simulink model "Vehicle_Dynamic_sim_V0605"  (R2017a)
settings: Solver=FixedStepAuto  StartTime=0.0  StopTime=50  FixedStep=0.001  RelTol=1e-3  EnableMultiTasking=on
PreLoadFcn:
  | load CarSim_FE4_2.mat
  | load Vehicle_information_test_0525_2017.mat
  | load CarSim0524.mat
values from neighbouring files (symbols this model uses):
  a = [(-2/tau - 1/tau_0) 1/tau 1/tau; 1/tau -2/tau 1/tau; 1/tau 1/tau -2/tau]    [MAE_272A_HW2_Q1a.m]    (also in Vehicle_Dynamic_main.m = 0.624; Vehicle_Dynamic_main_V0.m = 0.624; Vehicle_Dynamic_main_V01.m = 0.624; Vehicle_Dynamic_main_V0605.m = 0.624)
  aa = weight_front*wheelbase    (= 0.7875)    [Vehicle_Dynamic_main.m]    (also in Vehicle_Dynamic_main_V0.m; Vehicle_Dynamic_main_V01.m; Vehicle_Dynamic_main_V0605.m; Vehicle_Dynamic_main_V0629.m)
  b = [1/A 0; 0 1/A; 0 0]    [MAE_272A_HW2_Q1a.m]    (also in Vehicle_Dynamic_main.m = 0.624; Vehicle_Dynamic_main_V0.m = 0.624; Vehicle_Dynamic_main_V01.m = 0.624; Vehicle_Dynamic_main_V0605.m = 0.624)
  bb = weight_rear*wheelbase    (= 0.7875)    [Vehicle_Dynamic_main.m]    (also in Vehicle_Dynamic_main_V0.m; Vehicle_Dynamic_main_V01.m; Vehicle_Dynamic_main_V0605.m; Vehicle_Dynamic_main_V0629.m)
  g = 9.81    [Vehicle_Dynamic_main.m]    (also in Vehicle_Dynamic_main_V0.m; Vehicle_Dynamic_main_V01.m; Vehicle_Dynamic_main_V0605.m; Vehicle_Dynamic_main_V0629.m)
  hf = 0.20729    [Vehicle_Dynamic_main.m]    (also in Vehicle_Dynamic_main_V0.m; Vehicle_Dynamic_main_V01.m; Vehicle_Dynamic_main_V0605.m; Vehicle_Dynamic_main_V0629.m)
  hr = 0.20729    [Vehicle_Dynamic_main.m]    (also in Vehicle_Dynamic_main_V0.m; Vehicle_Dynamic_main_V01.m; Vehicle_Dynamic_main_V0605.m; Vehicle_Dynamic_main_V0629.m)
  initial_1 = [0 0 0 0]    [Vehicle_Dynamic_main.m]    (also in Vehicle_Dynamic_main_V0.m; Vehicle_Dynamic_main_V01.m; Vehicle_Dynamic_main_V0605.m; Vehicle_Dynamic_main_V0629.m)
  initial_2 = [0 0 0 0 (mf*g*weight_left/k_springf) (mf*g*weight_right/k_springf) ((mf*weight_left+mt)*g/k_tire_l) ((mf*weight_right+mt)*g/k_tire_r) 0]    [Vehicle_Dynamic_main.m]    (also in Vehicle_Dynamic_main_V0.m; Vehicle_Dynamic_main_V01.m; Vehicle_Dynamic_main_V0605.m; Vehicle_Dynamic_main_V0629.m)
  initial_3 = [0 0 0 0 (mr*g*weight_left/k_springr) (mr*g*weight_right/k_springr) ((mr*weight_left+mt)*g/k_tire_l) ((mr*weight_right+mt)*g/k_tire_r) 0]    [Vehicle_Dynamic_main.m]    (also in Vehicle_Dynamic_main_V0.m; Vehicle_Dynamic_main_V01.m; Vehicle_Dynamic_main_V0605.m; Vehicle_Dynamic_main_V0629.m)
  Izz = 89.99    [Vehicle_Dynamic_main.m]    (also in Vehicle_Dynamic_main_V0.m; Vehicle_Dynamic_main_V01.m; Vehicle_Dynamic_main_V0605.m; Vehicle_Dynamic_main_V0629.m)
  jf = mf*r_gy^2    (= 97.205445)    [Vehicle_Dynamic_main.m]    (also in Vehicle_Dynamic_main_V0.m; Vehicle_Dynamic_main_V01.m; Vehicle_Dynamic_main_V0605.m; Vehicle_Dynamic_main_V0629.m = 79.88796)
  jr = mr*r_gy^2    (= 97.205445)    [Vehicle_Dynamic_main.m]    (also in Vehicle_Dynamic_main_V0.m; Vehicle_Dynamic_main_V01.m; Vehicle_Dynamic_main_V0605.m; Vehicle_Dynamic_main_V0629.m = 79.88796)
  k_springf = 16640    [Vehicle_Dynamic_main.m]    (also in Vehicle_Dynamic_main_V0.m; Vehicle_Dynamic_main_V01.m; Vehicle_Dynamic_main_V0605.m; Vehicle_Dynamic_main_V0629.m = 13591.65)
  k_springr = 16640    [Vehicle_Dynamic_main.m]    (also in Vehicle_Dynamic_main_V0.m; Vehicle_Dynamic_main_V01.m; Vehicle_Dynamic_main_V0605.m; Vehicle_Dynamic_main_V0629.m = 13907.525)
  k_tire_l = 128571.4    [Vehicle_Dynamic_main.m]    (also in Vehicle_Dynamic_main_V0.m; Vehicle_Dynamic_main_V01.m; Vehicle_Dynamic_main_V0605.m; Vehicle_Dynamic_main_V0629.m)
  k_tire_r = 128571.4    [Vehicle_Dynamic_main.m]    (also in Vehicle_Dynamic_main_V0.m; Vehicle_Dynamic_main_V01.m; Vehicle_Dynamic_main_V0605.m; Vehicle_Dynamic_main_V0629.m)
  m_total = 237.6 + 70    (= 307.6)    [Vehicle_Dynamic_main.m]    (also in Vehicle_Dynamic_main_V0.m; Vehicle_Dynamic_main_V01.m; Vehicle_Dynamic_main_V0605.m; Vehicle_Dynamic_main_V0629.m = 252.8)
  mf = m_total*weight_front    (= 153.8)    [Vehicle_Dynamic_main.m]    (also in Vehicle_Dynamic_main_V0.m; Vehicle_Dynamic_main_V01.m; Vehicle_Dynamic_main_V0605.m; Vehicle_Dynamic_main_V0629.m = 126.4)
  mr = m_total*weight_rear    (= 153.8)    [Vehicle_Dynamic_main.m]    (also in Vehicle_Dynamic_main_V0.m; Vehicle_Dynamic_main_V01.m; Vehicle_Dynamic_main_V0605.m; Vehicle_Dynamic_main_V0629.m = 126.4)
  mt = 27.4/2    (= 13.7)    [Vehicle_Dynamic_main.m]    (also in Vehicle_Dynamic_main_V0.m; Vehicle_Dynamic_main_V01.m; Vehicle_Dynamic_main_V0605.m; Vehicle_Dynamic_main_V0629.m)
  r_damperf = 1416.7    [Vehicle_Dynamic_main.m]    (also in Vehicle_Dynamic_main_V0.m; Vehicle_Dynamic_main_V01.m; Vehicle_Dynamic_main_V0605.m; Vehicle_Dynamic_main_V0629.m = 5000)
  r_damperr = 1416.7    [Vehicle_Dynamic_main.m]    (also in Vehicle_Dynamic_main_V0.m; Vehicle_Dynamic_main_V01.m; Vehicle_Dynamic_main_V0605.m; Vehicle_Dynamic_main_V0629.m = 1428.6)
  sp_max = 30    [Vehicle_Dynamic_main.m]    (also in Vehicle_Dynamic_main_V0.m; Vehicle_Dynamic_main_V01.m; Vehicle_Dynamic_main_V0605.m; Vehicle_Dynamic_main_V0629.m)
  Tire_data_1 = [0	10.16645	30.135844	49.972681	69.612462	88.995136	108.063766	126.765417	145.053829	162.887632	180.230352	197.053076	213.331781	229.048232	244.189973	258.748997	272.722636	286.111778	298.921762	311.160594	322.839396	333.970622	344.56984	354.653955	364.239424	373.34582	381.991381	390.195233	397.976949	405.355211	412.349148	418.976995	425.256992	431.206487	436.841937	442.179356	447.234758	452.02326 ...(+3067 chars)    [Vehicle_Dynamic_main.m]    (also in Vehicle_Dynamic_main_V0.m; Vehicle_Dynamic_main_V01.m; Vehicle_Dynamic_main_V0605.m; Vehicle_Dynamic_main_V0629.m)
  track = 1.248    [Vehicle_Dynamic_main.m]    (also in Vehicle_Dynamic_main_V0.m; Vehicle_Dynamic_main_V01.m; Vehicle_Dynamic_main_V0605.m; Vehicle_Dynamic_main_V0629.m)
(part 1 of 2)
settings Model: Creator=Ping  LastModifiedBy=Ping
settings DataIOCC: ExternalInput=CarSim_FE4_2.getElement(1),CarSim_FE4_2.getElement(2)  LoadExternalInput=on
settings OptimizationCC: LifeSpan=inf
settings DebuggingCC: AlgebraicLoopMsg=error  SFUnexpectedBacktrackingDiag=warning  SFNoUnconditionalDefaultTransitionDiag=warning  SFExecutionAtInitializationDiag=none
settings GRTTargetCC: TargetLangStandard=C89/C90 (ANSI)  GeneratePreprocessorConditionals=Disable all
settings ConfigComp: CovMetricSettings=dw  CovHtmlReporting=on  CovSaveCumulativeToWorkspaceVar=on  CovSaveSingleToWorkspaceVar=on  CovExternalEMLEnable=off

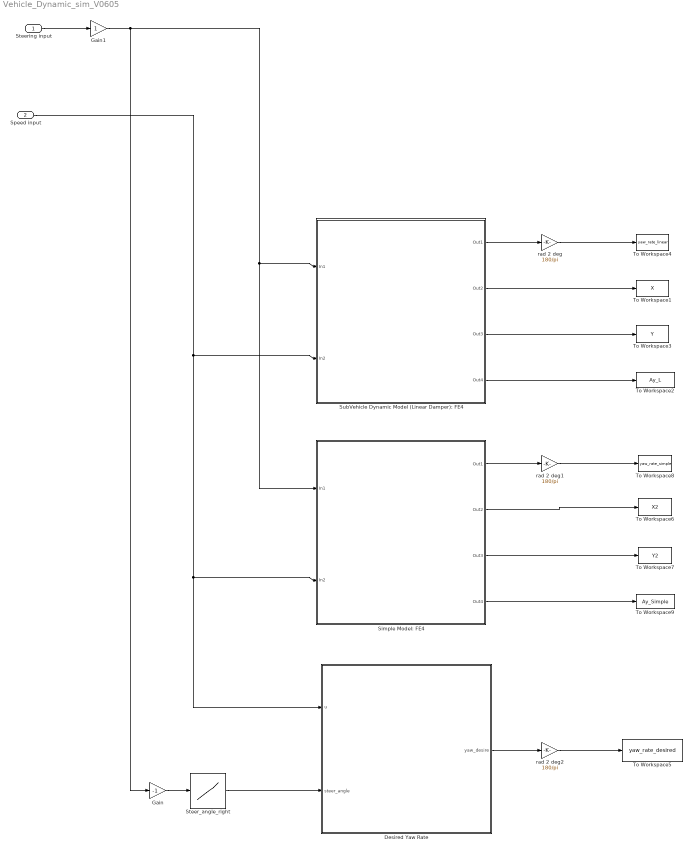
== system Vehicle_Dynamic_sim_V0605 ==
  Steering input : Inport
  Speed input : Inport  Port=2
  Desired Yaw Rate : MATLAB Function  TreatAsAtomicUnit=on
  Gain : Gain  Gain=-1
  Gain1 : Gain
  Simple Model: FE4 : Subsystem
  Steer_angle_right : Lookup_n-D  NumberOfTableDimensions=1  BreakpointsForDimension1=|  Table=|  InternalRulePriority=Speed  RndMeth=Simplest  InputSameDT=on
      BreakpointsForDimension1=|
      | [0
      | 0.014331519
      | 0.057018697
      | 0.127600467
      | 0.225615761
      | 0.350603511
      | 0.50210265
      | 0.679652108
      | 0.882790819
      | 1.111057714
      | 1.363991726
      | 1.64113179
      | 1.942016843
      | 2.266185824
      | 2.613177679
      | 2.982531359
      | 3.373785821
      | 3.786480036
      | 4.220152983
      | 4.674343657
      | 5.148591068
      | 5.642434246
      | 6.155412241
      | 6.687064127
      | 7.236929001
      | 7.804545991
      | 8.389454253
      | 8.991192974
      | 9.609301375
      | 10.24331871
      | 10.89278428
      | 11.55723741
      | 12.23621746
      | 12.92926384
      | 13.63591601
      | 14.35571344
      | 15.08819567
      | 15.83290225
      | 16.58937279
      | 17.35714693
      | 18.13576436
      | 18.92476478
      | 19.72368794
      | 20.53207362
      | 21.34946163
      | 22.17539181
      | 23.00940402
      | 23.85103814
      | 24.69983409
      | 25.55533177
      | 26.41707113
      | 27.28459211
      | 28.15743467
      | 29.03513874
      | 29.91724429
      | 30.80329126
      | 31.69281959
      | 32.5853692
      | 33.48047999
      | 34.37769185
      | 35.27654463
      | 36.17657814
      | 37.07733217
      | 37.97834646
      | 38.87916071
      | 39.77931454
      | 40.67834756
      | 41.57579927
      | 42.47120913
      | 43.36411653
      | 44.25406075
      | 45.14058103
      | 46.0232165
      | 46.90150619
      | 47.77498904
      | 48.6432039
      | 49.5056895
      | 50.36198444
      | 51.21162725
      | 52.05415631
      | 52.88910986
      | 53.71602605
      | 54.53444287
      | 55.3438982
      | 56.14392975
      | 56.93407511
      | 57.71387173
      | 58.48285692
      | 59.24056782
      | 59.98654144
      | 60.72031464
      | 61.44142415
      | 62.14940652
      | 62.84379819
      | 63.52413542
      | 64.18995437
      | 64.84079103
      | 65.47618129
      | 66.09566087
      | 66.6987654
      | 67.28503038
      | 67.85399122
      | 68.4051832
      | 68.93814154
      | 69.45240136
      | 69.94749771
      | 70.4229656
      | 70.87833997
      | 71.31315575
      | 71.72694784
      | 72.11925116
      | 72.48960062
      | 72.83753118
      | 73.16257784
      | 73.46427569
      | 73.74215988
      | 73.9957657
      | 74.22462855
      | 74.42828398
      | 74.60626772
      | 74.75811568
      | 74.883364
      | 74.98154904
      | 75.0522074
      | 75.09487599
      | 75.10909199
      | ]
      Table=|
      | [0.0000
      | -0.0046
      | -0.0183
      | -0.0409
      | -0.0723
      | -0.1124
      | -0.1609
      | -0.2178
      | -0.2828
      | -0.3559
      | -0.4369
      | -0.5255
      | -0.6218
      | -0.7254
      | -0.8364
      | -0.9544
      | -1.0793
      | -1.2110
      | -1.3494
      | -1.4943
      | -1.6454
      | -1.8028
      | -1.9661
      | -2.1353
      | -2.3102
      | -2.4907
      | -2.6765
      | -2.8676
      | -3.0638
      | -3.2649
      | -3.4708
      | -3.6813
      | -3.8963
      | -4.1157
      | -4.3392
      | -4.5668
      | -4.7982
      | -5.0334
      | -5.2721
      | -5.5144
      | -5.7599
      | -6.0085
      | -6.2602
      | -6.5147
      | -6.7720
      | -7.0318
      | -7.2941
      | -7.5586
      | -7.8254
      | -8.0941
      | -8.3647
      | -8.6370
      | -8.9109
      | -9.1862
      | -9.4629
      | -9.7407
      | -10.0196
      | -10.2993
      | -10.5799
      | -10.8610
      | -11.1426
      | -11.4246
      | -11.7067
      | -11.9890
      | -12.2711
      | -12.5531
      | -12.8347
      | -13.1158
      | -13.3963
      | -13.6761
      | -13.9549
      | -14.2327
      | -14.5094
      | -14.7847
      | -15.0586
      | -15.3309
      | -15.6015
      | -15.8701
      | -16.1368
      | -16.4013
      | -16.6636
      | -16.9234
      | -17.1806
      | -17.4350
      | -17.6867
      | -17.9353
      | -18.1807
      | -18.4229
      | -18.6616
      | -18.8967
      | -19.1281
      | -19.3555
      | -19.5790
      | -19.7982
      | -20.0132
      | -20.2236
      | -20.4294
      | -20.6304
      | -20.8265
      | -21.0175
      | -21.2032
      | -21.3836
      | -21.5584
      | -21.7275
      | -21.8908
      | -22.0480
      | -22.1991
      | -22.3438
      | -22.4821
      | -22.6138
      | -22.7386
      | -22.8566
      | -22.9674
      | -23.0710
      | -23.1672
      | -23.2558
      | -23.3367
      | -23.4098
      | -23.4748
      | -23.5317
      | -23.5802
      | -23.6203
      | -23.6517
      | -23.6744
      | -23.6881
      | -23.6928
      | ]
  SubVehicle Dynamic Model (Linear Damper): FE4 : Subsystem
  To Workspace1 : ToWorkspace  VariableName=X  SaveFormat=Timeseries  SampleTime=-1
  To Workspace2 : ToWorkspace  VariableName=Ay_L  SaveFormat=Timeseries  SampleTime=-1
  To Workspace3 : ToWorkspace  VariableName=Y  SaveFormat=Timeseries  SampleTime=-1
  To Workspace4 : ToWorkspace  VariableName=yaw_rate_linear  SaveFormat=Timeseries  SampleTime=-1
  To Workspace5 : ToWorkspace  VariableName=yaw_rate_desired  SaveFormat=Timeseries  SampleTime=-1
  To Workspace6 : ToWorkspace  VariableName=X2  SaveFormat=Timeseries  SampleTime=-1
  To Workspace7 : ToWorkspace  VariableName=Y2  SaveFormat=Timeseries  SampleTime=-1
  To Workspace8 : ToWorkspace  VariableName=yaw_rate_simple  SaveFormat=Timeseries  SampleTime=-1
  To Workspace9 : ToWorkspace  VariableName=Ay_Simple  SaveFormat=Timeseries  SampleTime=-1
  rad 2 deg : Gain  Gain=180/pi
  rad 2 deg1 : Gain  Gain=180/pi
  rad 2 deg2 : Gain  Gain=180/pi
  wires:
  SubVehicle Dynamic Model (Linear Damper): FE4/1(Out1) -> rad 2 deg/1
  SubVehicle Dynamic Model (Linear Damper): FE4/2(Out2) -> To Workspace1/1
  SubVehicle Dynamic Model (Linear Damper): FE4/3(Out3) -> To Workspace3/1
  Simple Model: FE4/2(Out2) -> To Workspace6/1
  Simple Model: FE4/3(Out3) -> To Workspace7/1
  Simple Model: FE4/1(Out1) -> rad 2 deg1/1
  Speed input/1 -> Desired Yaw Rate/1(u), Simple Model: FE4/2(In2), SubVehicle Dynamic Model (Linear Damper): FE4/2(In2)
  Desired Yaw Rate/1(yaw_desire) -> rad 2 deg2/1
  Steering input/1 -> Gain1/1
  Gain1/1 -> Gain/1, Simple Model: FE4/1(In1), SubVehicle Dynamic Model (Linear Damper): FE4/1(In1)
  Steer_angle_right/1 -> Desired Yaw Rate/2(steer_angle)
  Gain/1 -> Steer_angle_right/1
  rad 2 deg/1 -> To Workspace4/1
  rad 2 deg1/1 -> To Workspace8/1
  rad 2 deg2/1 -> To Workspace5/1
  SubVehicle Dynamic Model (Linear Damper): FE4/4(Out4) -> To Workspace2/1
  Simple Model: FE4/4(Out4) -> To Workspace9/1

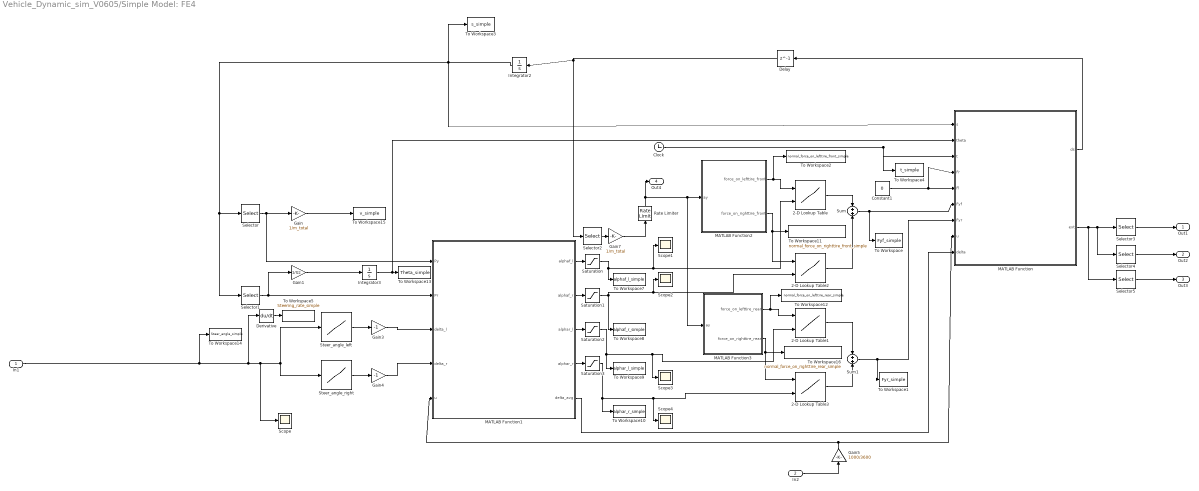
== system Vehicle_Dynamic_sim_V0605/Simple Model: FE4 ==
  In1 : Inport
  In2 : Inport  Port=2
  2-D Lookup Table{,1..3} (4 alike) : Lookup_n-D  BreakpointsForDimension1=[222.41,667.23,1112.06]  BreakpointsForDimension2=[0,0.001745328,0.003490656,0.005235983,0.006981311,0.008726639,0.010471967,0.012217294,0.013962622,0.01570795,0.017453278,0.019198606,0.020943933,0.022689261,0.024434589,0.026179917,0.027925244,0.029670572,0.0314159,0.033161228,0.034906556,0.036651883,0.038397211,0.040142539,0.041887867,0.043633194,0.045378522,0.04712385,0.048869178,0.050614506,0.052359833,0.054105161,0.055850489,0.057595817,0.059341144,0.061086472,0.0628318,0.064577128,0.066322456,0.068067783,0.069813111,0.071558439,0.073303767,0.075049094,0.076794422,0.07853975,0.080285078,0.082030406,0.083775733,0.085521061,0.087266389,0.089011717,0.090757044,0.092502372,0.0942477,0.095993028,0.097738356,0.099483683,0.101229011,0.102974339,0.104719667,0.106464994,0.108210322,0.10995565,0.111700978,0.113446306,0.115191633,0.116936961,0.118682289,0.120427617,0.122172944,0.123918272,0.1256636,0.127408928,0.129154256,0.130899583,0.132644911,0.134390239,0.136135567,0.137880894,0.139626222,0.14137155,0.143116878,0.144862206,0.146607533,0.148352861,0.150098189,0.151843517,0.153588844,0.155334172,0.1570795,0.158824828,0.160570156,0.162315483,0.164060811,0.165806139,0.167551467,0.169296794,0.171042122,0.17278745,0.174532778,0.176278106]  Table=Tire_data_1  InternalRulePriority=Speed  RndMeth=Simplest  InputSameDT=on
  Clock : Clock
  Constant1 : Constant  Value=0
  Delay : Delay  DelayLength=1  InitialCondition=0  SampleTime=0.001
  Derivative : Derivative
  Gain : Gain  Gain=1/m_total
      settings: AttributesFormatString=%<Gain>
  Gain1 : Gain  Gain=1/Izz
      settings: AttributesFormatString=%<Gain>
  Gain3 : Gain  Gain=-1
      settings: AttributesFormatString=%<Gain>
  Gain4 : Gain  Gain=-1
      settings: AttributesFormatString=%<Gain>
  Gain5 : Gain  Gain=1000/3600
  Gain7 : Gain  Gain=1/m_total
      settings: AttributesFormatString=%<Gain>
  Integrator2 : Integrator  InitialCondition=initial_1  UpperSaturationLimit=50000  LowerSaturationLimit=-50000
  Integrator3 : Integrator
  MATLAB Function : MATLAB Function  TreatAsAtomicUnit=on
  MATLAB Function1 : MATLAB Function  TreatAsAtomicUnit=on
  MATLAB Function2 : MATLAB Function  TreatAsAtomicUnit=on
  MATLAB Function3 : MATLAB Function  TreatAsAtomicUnit=on
  Rate Limiter : RateLimiter  RisingSlewLimit=10  FallingSlewLimit=-10  SampleTimeMode=inherited
  Saturation{,1..3} (4 alike) : Saturate  UpperLimit=sp_max  LowerLimit=-sp_max
  Scope{,1..4} (5 alike) : Scope
  Selector : Selector  InputPortWidth=4  IndexOptions=Index vector (dialog)  Indices=[1]  OutputSizes=1
  Selector1 : Selector  InputPortWidth=4  IndexOptions=Index vector (dialog)  Indices=[2]  OutputSizes=1
  Selector2 : Selector  InputPortWidth=4  IndexOptions=Index vector (dialog)  Indices=[1]  OutputSizes=1
  Selector3 : Selector  InputPortWidth=3  IndexOptions=Index vector (dialog)  Indices=[1]  OutputSizes=1
  Selector4 : Selector  InputPortWidth=3  IndexOptions=Index vector (dialog)  Indices=[2]  OutputSizes=1
  Selector5 : Selector  InputPortWidth=3  IndexOptions=Index vector (dialog)  Indices=[3]  OutputSizes=1
  Steer_angle_left : Lookup_n-D  NumberOfTableDimensions=1  BreakpointsForDimension1=|  Table=|  InternalRulePriority=Speed  RndMeth=Simplest  InputSameDT=on
      BreakpointsForDimension1=|
      | [0
      | 0.014331519
      | 0.057018697
      | 0.127600467
      | 0.225615761
      | 0.350603511
      | 0.50210265
      | 0.679652108
      | 0.882790819
      | 1.111057714
      | 1.363991726
      | 1.64113179
      | 1.942016843
      | 2.266185824
      | 2.613177679
      | 2.982531359
      | 3.373785821
      | 3.786480036
      | 4.220152983
      | 4.674343657
      | 5.148591068
      | 5.642434246
      | 6.155412241
      | 6.687064127
      | 7.236929001
      | 7.804545991
      | 8.389454253
      | 8.991192974
      | 9.609301375
      | 10.24331871
      | 10.89278428
      | 11.55723741
      | 12.23621746
      | 12.92926384
      | 13.63591601
      | 14.35571344
      | 15.08819567
      | 15.83290225
      | 16.58937279
      | 17.35714693
      | 18.13576436
      | 18.92476478
      | 19.72368794
      | 20.53207362
      | 21.34946163
      | 22.17539181
      | 23.00940402
      | 23.85103814
      | 24.69983409
      | 25.55533177
      | 26.41707113
      | 27.28459211
      | 28.15743467
      | 29.03513874
      | 29.91724429
      | 30.80329126
      | 31.69281959
      | 32.5853692
      | 33.48047999
      | 34.37769185
      | 35.27654463
      | 36.17657814
      | 37.07733217
      | 37.97834646
      | 38.87916071
      | 39.77931454
      | 40.67834756
      | 41.57579927
      | 42.47120913
      | 43.36411653
      | 44.25406075
      | 45.14058103
      | 46.0232165
      | 46.90150619
      | 47.77498904
      | 48.6432039
      | 49.5056895
      | 50.36198444
      | 51.21162725
      | 52.05415631
      | 52.88910986
      | 53.71602605
      | 54.53444287
      | 55.3438982
      | 56.14392975
      | 56.93407511
      | 57.71387173
      | 58.48285692
      | 59.24056782
      | 59.98654144
      | 60.72031464
      | 61.44142415
      | 62.14940652
      | 62.84379819
      | 63.52413542
      | 64.18995437
      | 64.84079103
      | 65.47618129
      | 66.09566087
      | 66.6987654
      | 67.28503038
      | 67.85399122
      | 68.4051832
      | 68.93814154
      | 69.45240136
      | 69.94749771
      | 70.4229656
      | 70.87833997
      | 71.31315575
      | 71.72694784
      | 72.11925116
      | 72.48960062
      | 72.83753118
      | 73.16257784
      | 73.46427569
      | 73.74215988
      | 73.9957657
      | 74.22462855
      | 74.42828398
      | 74.60626772
      | 74.75811568
      | 74.883364
      | 74.98154904
      | 75.0522074
      | 75.09487599
      | 75.10909199
      | ]
      Table=|
      | [0.0000
      | -0.0046
      | -0.0183
      | -0.0409
      | -0.0723
      | -0.1124
      | -0.1610
      | -0.2180
      | -0.2831
      | -0.3564
      | -0.4376
      | -0.5266
      | -0.6233
      | -0.7275
      | -0.8391
      | -0.9579
      | -1.0838
      | -1.2167
      | -1.3565
      | -1.5029
      | -1.6559
      | -1.8154
      | -1.9811
      | -2.1531
      | -2.3310
      | -2.5148
      | -2.7045
      | -2.8997
      | -3.1005
      | -3.3066
      | -3.5180
      | -3.7344
      | -3.9559
      | -4.1822
      | -4.4133
      | -4.6489
      | -4.8890
      | -5.1334
      | -5.3821
      | -5.6348
      | -5.8915
      | -6.1519
      | -6.4161
      | -6.6839
      | -6.9551
      | -7.2295
      | -7.5072
      | -7.7879
      | -8.0715
      | -8.3579
      | -8.6470
      | -8.9386
      | -9.2326
      | -9.5289
      | -9.8272
      | -10.1276
      | -10.4299
      | -10.7338
      | -11.0394
      | -11.3464
      | -11.6547
      | -11.9642
      | -12.2748
      | -12.5863
      | -12.8985
      | -13.2113
      | -13.5246
      | -13.8382
      | -14.1519
      | -14.4657
      | -14.7794
      | -15.0928
      | -15.4057
      | -15.7180
      | -16.0296
      | -16.3403
      | -16.6498
      | -16.9582
      | -17.2651
      | -17.5704
      | -17.8739
      | -18.1755
      | -18.4750
      | -18.7722
      | -19.0669
      | -19.3589
      | -19.6481
      | -19.9342
      | -20.2170
      | -20.4964
      | -20.7722
      | -21.0441
      | -21.3119
      | -21.5755
      | -21.8345
      | -22.0889
      | -22.3383
      | -22.5826
      | -22.8216
      | -23.0549
      | -23.2825
      | -23.5040
      | -23.7192
      | -23.9279
      | -24.1298
      | -24.3247
      | -24.5125
      | -24.6927
      | -24.8653
      | -25.0299
      | -25.1863
      | -25.3343
      | -25.4736
      | -25.6040
      | -25.7253
      | -25.8372
      | -25.9395
      | -26.0319
      | -26.1142
      | -26.1863
      | -26.2478
      | -26.2986
      | -26.3385
      | -26.3672
      | -26.3845
      | -26.3903
      | ]
  Steer_angle_right : Lookup_n-D  NumberOfTableDimensions=1  BreakpointsForDimension1=|  Table=|  InternalRulePriority=Speed  RndMeth=Simplest  InputSameDT=on
      BreakpointsForDimension1=|
      | [0
      | 0.014331519
      | 0.057018697
      | 0.127600467
      | 0.225615761
      | 0.350603511
      | 0.50210265
      | 0.679652108
      | 0.882790819
      | 1.111057714
      | 1.363991726
      | 1.64113179
      | 1.942016843
      | 2.266185824
      | 2.613177679
      | 2.982531359
      | 3.373785821
      | 3.786480036
      | 4.220152983
      | 4.674343657
      | 5.148591068
      | 5.642434246
      | 6.155412241
      | 6.687064127
      | 7.236929001
      | 7.804545991
      | 8.389454253
      | 8.991192974
      | 9.609301375
      | 10.24331871
      | 10.89278428
      | 11.55723741
      | 12.23621746
      | 12.92926384
      | 13.63591601
      | 14.35571344
      | 15.08819567
      | 15.83290225
      | 16.58937279
      | 17.35714693
      | 18.13576436
      | 18.92476478
      | 19.72368794
      | 20.53207362
      | 21.34946163
      | 22.17539181
      | 23.00940402
      | 23.85103814
      | 24.69983409
      | 25.55533177
      | 26.41707113
      | 27.28459211
      | 28.15743467
      | 29.03513874
      | 29.91724429
      | 30.80329126
      | 31.69281959
      | 32.5853692
      | 33.48047999
      | 34.37769185
      | 35.27654463
      | 36.17657814
      | 37.07733217
      | 37.97834646
      | 38.87916071
      | 39.77931454
      | 40.67834756
      | 41.57579927
      | 42.47120913
      | 43.36411653
      | 44.25406075
      | 45.14058103
      | 46.0232165
      | 46.90150619
      | 47.77498904
      | 48.6432039
      | 49.5056895
      | 50.36198444
      | 51.21162725
      | 52.05415631
      | 52.88910986
      | 53.71602605
      | 54.53444287
      | 55.3438982
      | 56.14392975
      | 56.93407511
      | 57.71387173
      | 58.48285692
      | 59.24056782
      | 59.98654144
      | 60.72031464
      | 61.44142415
      | 62.14940652
      | 62.84379819
      | 63.52413542
      | 64.18995437
      | 64.84079103
      | 65.47618129
      | 66.09566087
      | 66.6987654
      | 67.28503038
      | 67.85399122
      | 68.4051832
      | 68.93814154
      | 69.45240136
      | 69.94749771
      | 70.4229656
      | 70.87833997
      | 71.31315575
      | 71.72694784
      | 72.11925116
      | 72.48960062
      | 72.83753118
      | 73.16257784
      | 73.46427569
      | 73.74215988
      | 73.9957657
      | 74.22462855
      | 74.42828398
      | 74.60626772
      | 74.75811568
      | 74.883364
      | 74.98154904
      | 75.0522074
      | 75.09487599
      | 75.10909199
      | ]
      Table=|
      | [0.0000
      | -0.0046
      | -0.0183
      | -0.0409
      | -0.0723
      | -0.1124
      | -0.1609
      | -0.2178
      | -0.2828
      | -0.3559
      | -0.4369
      | -0.5255
      | -0.6218
      | -0.7254
      | -0.8364
      | -0.9544
      | -1.0793
      | -1.2110
      | -1.3494
      | -1.4943
      | -1.6454
      | -1.8028
      | -1.9661
      | -2.1353
      | -2.3102
      | -2.4907
      | -2.6765
      | -2.8676
      | -3.0638
      | -3.2649
      | -3.4708
      | -3.6813
      | -3.8963
      | -4.1157
      | -4.3392
      | -4.5668
      | -4.7982
      | -5.0334
      | -5.2721
      | -5.5144
      | -5.7599
      | -6.0085
      | -6.2602
      | -6.5147
      | -6.7720
      | -7.0318
      | -7.2941
      | -7.5586
      | -7.8254
      | -8.0941
      | -8.3647
      | -8.6370
      | -8.9109
      | -9.1862
      | -9.4629
      | -9.7407
      | -10.0196
      | -10.2993
      | -10.5799
      | -10.8610
      | -11.1426
      | -11.4246
      | -11.7067
      | -11.9890
      | -12.2711
      | -12.5531
      | -12.8347
      | -13.1158
      | -13.3963
      | -13.6761
      | -13.9549
      | -14.2327
      | -14.5094
      | -14.7847
      | -15.0586
      | -15.3309
      | -15.6015
      | -15.8701
      | -16.1368
      | -16.4013
      | -16.6636
      | -16.9234
      | -17.1806
      | -17.4350
      | -17.6867
      | -17.9353
      | -18.1807
      | -18.4229
      | -18.6616
      | -18.8967
      | -19.1281
      | -19.3555
      | -19.5790
      | -19.7982
      | -20.0132
      | -20.2236
      | -20.4294
      | -20.6304
      | -20.8265
      | -21.0175
      | -21.2032
      | -21.3836
      | -21.5584
      | -21.7275
      | -21.8908
      | -22.0480
      | -22.1991
      | -22.3438
      | -22.4821
      | -22.6138
      | -22.7386
      | -22.8566
      | -22.9674
      | -23.0710
      | -23.1672
      | -23.2558
      | -23.3367
      | -23.4098
      | -23.4748
      | -23.5317
      | -23.5802
      | -23.6203
      | -23.6517
      | -23.6744
      | -23.6881
      | -23.6928
      | ]
  Sum : Sum
  Sum1 : Sum
  To Workspace : ToWorkspace  VariableName=Fyf_simple  SaveFormat=Timeseries  SampleTime=-1
  To Workspace1 : ToWorkspace  VariableName=Fyr_simple  SaveFormat=Timeseries  SampleTime=-1
  To Workspace10 : ToWorkspace  VariableName=alphar_r_simple  SaveFormat=Timeseries  SampleTime=-1
  To Workspace11 : ToWorkspace  VariableName=normal_force_on_righttire_front_simple  SaveFormat=Timeseries  SampleTime=-1
  To Workspace12 : ToWorkspace  VariableName=normal_force_on_lefttire_rear_simple  SaveFormat=Timeseries  SampleTime=-1
  To Workspace13 : ToWorkspace  VariableName=Theta_simple  SaveFormat=Timeseries  SampleTime=-1
  To Workspace14 : ToWorkspace  VariableName=Steer_angle_simple  SaveFormat=Timeseries  SampleTime=-1
  To Workspace15 : ToWorkspace  VariableName=v_simple  SaveFormat=Timeseries  SampleTime=-1
  To Workspace16 : ToWorkspace  VariableName=normal_force_on_righttire_rear_simple  SaveFormat=Timeseries  SampleTime=-1
  To Workspace2 : ToWorkspace  VariableName=normal_force_on_lefttire_front_simple  SaveFormat=Timeseries  SampleTime=-1
  To Workspace3 : ToWorkspace  VariableName=s_simple  SaveFormat=Timeseries  SampleTime=-1
  To Workspace4 : ToWorkspace  VariableName=t_simple  SaveFormat=Timeseries  SampleTime=-1
  To Workspace5 : ToWorkspace  VariableName=Steering_rate_simple  SaveFormat=Timeseries  SampleTime=-1
  To Workspace7 : ToWorkspace  VariableName=alphaf_l_simple  SaveFormat=Timeseries  SampleTime=-1
  To Workspace8 : ToWorkspace  VariableName=alphaf_r_simple  SaveFormat=Timeseries  SampleTime=-1
  To Workspace9 : ToWorkspace  VariableName=alphar_l_simple  SaveFormat=Timeseries  SampleTime=-1
  Out1 : Outport
  Out2 : Outport  Port=2
  Out3 : Outport  Port=3
  Out4 : Outport  Port=4
  wires:
  Saturation2/1 -> To Workspace9/1, Scope3/1, 2-D Lookup Table1/2
  MATLAB Function1/1(alphaf_l) -> Saturation/1
  MATLAB Function/2(ext) -> Selector5/1, Selector4/1, Selector3/1
  Steer_angle_right/1 -> Gain4/1
  Constant1/1 -> MATLAB Function/4(Fr), MATLAB Function/5(Fl)
  Derivative/1 -> To Workspace5/1
  MATLAB Function1/3(alphar_l) -> Saturation2/1
  Saturation/1 -> To Workspace7/1, Scope1/1, 2-D Lookup Table/2
  Gain1/1 -> Integrator3/1
  Selector/1 -> MATLAB Function1/1(Py), Gain/1
  Selector4/1 -> Out2/1
  Sum/1 -> To Workspace/1, MATLAB Function/6(Fyf)
  Steer_angle_left/1 -> Gain3/1
  In2/1 -> Gain5/1
  MATLAB Function2/2(force_on_righttire_front) -> To Workspace11/1, 2-D Lookup Table2/1
  2-D Lookup Table/1 -> Sum/1
  2-D Lookup Table2/1 -> Sum/2
  Selector5/1 -> Out3/1
  2-D Lookup Table3/1 -> Sum1/2
  Saturation1/1 -> To Workspace8/1, 2-D Lookup Table2/2, Scope2/1
  Delay/1 -> Selector2/1, Integrator2/1
  Integrator2/1 -> MATLAB Function/1(s), To Workspace3/1, Selector/1, Selector1/1
  Sum1/1 -> To Workspace1/1, MATLAB Function/7(Fyr)
  2-D Lookup Table1/1 -> Sum1/1
  MATLAB Function1/4(alphar_r) -> Saturation3/1
  Selector1/1 -> Gain1/1, MATLAB Function1/2(Pr)
  MATLAB Function3/1(force_on_lefttire_rear) -> To Workspace12/1, 2-D Lookup Table1/1
  Selector2/1 -> Gain7/1
  Integrator3/1 -> MATLAB Function/2(theta), To Workspace13/1
  MATLAB Function2/1(force_on_lefttire_front) -> To Workspace2/1, 2-D Lookup Table/1
  Clock/1 -> To Workspace4/1, MATLAB Function/3(t)
  MATLAB Function/1(ds) -> Delay/1
  Rate Limiter/1 -> Out4/1, MATLAB Function3/1(ay), MATLAB Function2/1(ay)
  Gain5/1 -> MATLAB Function/8(u), MATLAB Function1/5(u)
  Selector3/1 -> Out1/1
  MATLAB Function1/5(delta_avg) -> MATLAB Function/9(delta)
  Gain4/1 -> MATLAB Function1/4(delta_r)
  Gain/1 -> To Workspace15/1
  In1/1 -> To Workspace14/1, Derivative/1, Scope/1, Steer_angle_left/1, Steer_angle_right/1
  Gain3/1 -> MATLAB Function1/3(delta_l)
  MATLAB Function1/2(alphaf_r) -> Saturation1/1
  Saturation3/1 -> To Workspace10/1, Scope4/1, 2-D Lookup Table3/2
  MATLAB Function3/2(force_on_righttire_rear) -> To Workspace16/1, 2-D Lookup Table3/1
  Gain7/1 -> Rate Limiter/1

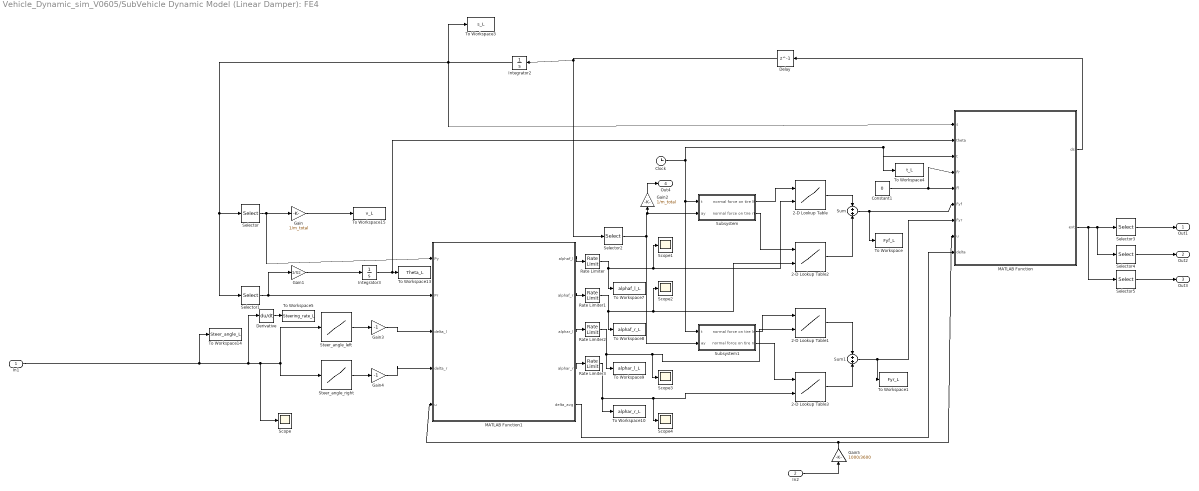
== system Vehicle_Dynamic_sim_V0605/SubVehicle Dynamic Model (Linear Damper): FE4 ==
  In1 : Inport
  In2 : Inport  Port=2
  2-D Lookup Table{,1..3} (4 alike) : Lookup_n-D  BreakpointsForDimension1=[222.41,667.23,1112.06]  BreakpointsForDimension2=[0,0.001745328,0.003490656,0.005235983,0.006981311,0.008726639,0.010471967,0.012217294,0.013962622,0.01570795,0.017453278,0.019198606,0.020943933,0.022689261,0.024434589,0.026179917,0.027925244,0.029670572,0.0314159,0.033161228,0.034906556,0.036651883,0.038397211,0.040142539,0.041887867,0.043633194,0.045378522,0.04712385,0.048869178,0.050614506,0.052359833,0.054105161,0.055850489,0.057595817,0.059341144,0.061086472,0.0628318,0.064577128,0.066322456,0.068067783,0.069813111,0.071558439,0.073303767,0.075049094,0.076794422,0.07853975,0.080285078,0.082030406,0.083775733,0.085521061,0.087266389,0.089011717,0.090757044,0.092502372,0.0942477,0.095993028,0.097738356,0.099483683,0.101229011,0.102974339,0.104719667,0.106464994,0.108210322,0.10995565,0.111700978,0.113446306,0.115191633,0.116936961,0.118682289,0.120427617,0.122172944,0.123918272,0.1256636,0.127408928,0.129154256,0.130899583,0.132644911,0.134390239,0.136135567,0.137880894,0.139626222,0.14137155,0.143116878,0.144862206,0.146607533,0.148352861,0.150098189,0.151843517,0.153588844,0.155334172,0.1570795,0.158824828,0.160570156,0.162315483,0.164060811,0.165806139,0.167551467,0.169296794,0.171042122,0.17278745,0.174532778,0.176278106]  Table=Tire_data_1  InternalRulePriority=Speed  RndMeth=Simplest  InputSameDT=on
  Clock : Clock
  Constant1 : Constant  Value=0
  Delay : Delay  DelayLength=1  InitialCondition=0  SampleTime=0.001
  Derivative : Derivative
  Gain : Gain  Gain=1/m_total
      settings: AttributesFormatString=%<Gain>
  Gain1 : Gain  Gain=1/Izz
      settings: AttributesFormatString=%<Gain>
  Gain2 : Gain  Gain=1/m_total
  Gain3 : Gain  Gain=-1
      settings: AttributesFormatString=%<Gain>
  Gain4 : Gain  Gain=-1
      settings: AttributesFormatString=%<Gain>
  Gain5 : Gain  Gain=1000/3600
  Integrator2 : Integrator  InitialCondition=initial_1
  Integrator3 : Integrator
  MATLAB Function : MATLAB Function  TreatAsAtomicUnit=on
  MATLAB Function1 : MATLAB Function  TreatAsAtomicUnit=on
  Rate Limiter{,1..3} (4 alike) : RateLimiter  RisingSlewLimit=5  FallingSlewLimit=-5  SampleTimeMode=inherited
  Scope{,1..4} (5 alike) : Scope
  Selector : Selector  InputPortWidth=4  IndexOptions=Index vector (dialog)  Indices=[1]  OutputSizes=1
  Selector1 : Selector  InputPortWidth=4  IndexOptions=Index vector (dialog)  Indices=[2]  OutputSizes=1
  Selector2 : Selector  InputPortWidth=4  IndexOptions=Index vector (dialog)  Indices=[1]  OutputSizes=1
  Selector3 : Selector  InputPortWidth=3  IndexOptions=Index vector (dialog)  Indices=[1]  OutputSizes=1
  Selector4 : Selector  InputPortWidth=3  IndexOptions=Index vector (dialog)  Indices=[2]  OutputSizes=1
  Selector5 : Selector  InputPortWidth=3  IndexOptions=Index vector (dialog)  Indices=[3]  OutputSizes=1
  Steer_angle_left : Lookup_n-D  NumberOfTableDimensions=1  BreakpointsForDimension1=|  Table=|  InternalRulePriority=Speed  RndMeth=Simplest  InputSameDT=on
      BreakpointsForDimension1=|
      | [0
      | 0.014331519
      | 0.057018697
      | 0.127600467
      | 0.225615761
      | 0.350603511
      | 0.50210265
      | 0.679652108
      | 0.882790819
      | 1.111057714
      | 1.363991726
      | 1.64113179
      | 1.942016843
      | 2.266185824
      | 2.613177679
      | 2.982531359
      | 3.373785821
      | 3.786480036
      | 4.220152983
      | 4.674343657
      | 5.148591068
      | 5.642434246
      | 6.155412241
      | 6.687064127
      | 7.236929001
      | 7.804545991
      | 8.389454253
      | 8.991192974
      | 9.609301375
      | 10.24331871
      | 10.89278428
      | 11.55723741
      | 12.23621746
      | 12.92926384
      | 13.63591601
      | 14.35571344
      | 15.08819567
      | 15.83290225
      | 16.58937279
      | 17.35714693
      | 18.13576436
      | 18.92476478
      | 19.72368794
      | 20.53207362
      | 21.34946163
      | 22.17539181
      | 23.00940402
      | 23.85103814
      | 24.69983409
      | 25.55533177
      | 26.41707113
      | 27.28459211
      | 28.15743467
      | 29.03513874
      | 29.91724429
      | 30.80329126
      | 31.69281959
      | 32.5853692
      | 33.48047999
      | 34.37769185
      | 35.27654463
      | 36.17657814
      | 37.07733217
      | 37.97834646
      | 38.87916071
      | 39.77931454
      | 40.67834756
      | 41.57579927
      | 42.47120913
      | 43.36411653
      | 44.25406075
      | 45.14058103
      | 46.0232165
      | 46.90150619
      | 47.77498904
      | 48.6432039
      | 49.5056895
      | 50.36198444
      | 51.21162725
      | 52.05415631
      | 52.88910986
      | 53.71602605
      | 54.53444287
      | 55.3438982
      | 56.14392975
      | 56.93407511
      | 57.71387173
      | 58.48285692
      | 59.24056782
      | 59.98654144
      | 60.72031464
      | 61.44142415
      | 62.14940652
      | 62.84379819
      | 63.52413542
      | 64.18995437
      | 64.84079103
      | 65.47618129
      | 66.09566087
      | 66.6987654
      | 67.28503038
      | 67.85399122
      | 68.4051832
      | 68.93814154
      | 69.45240136
      | 69.94749771
      | 70.4229656
      | 70.87833997
      | 71.31315575
      | 71.72694784
      | 72.11925116
      | 72.48960062
      | 72.83753118
      | 73.16257784
      | 73.46427569
      | 73.74215988
      | 73.9957657
      | 74.22462855
      | 74.42828398
      | 74.60626772
      | 74.75811568
      | 74.883364
      | 74.98154904
      | 75.0522074
      | 75.09487599
      | 75.10909199
      | ]
      Table=|
      | [0.0000
      | -0.0046
      | -0.0183
      | -0.0409
      | -0.0723
      | -0.1124
      | -0.1610
      | -0.2180
      | -0.2831
      | -0.3564
      | -0.4376
      | -0.5266
      | -0.6233
      | -0.7275
      | -0.8391
      | -0.9579
      | -1.0838
      | -1.2167
      | -1.3565
      | -1.5029
      | -1.6559
      | -1.8154
      | -1.9811
      | -2.1531
      | -2.3310
      | -2.5148
      | -2.7045
      | -2.8997
      | -3.1005
      | -3.3066
      | -3.5180
      | -3.7344
      | -3.9559
      | -4.1822
      | -4.4133
      | -4.6489
      | -4.8890
      | -5.1334
      | -5.3821
      | -5.6348
      | -5.8915
      | -6.1519
      | -6.4161
      | -6.6839
      | -6.9551
      | -7.2295
      | -7.5072
      | -7.7879
      | -8.0715
      | -8.3579
      | -8.6470
      | -8.9386
      | -9.2326
      | -9.5289
      | -9.8272
      | -10.1276
      | -10.4299
      | -10.7338
      | -11.0394
      | -11.3464
      | -11.6547
      | -11.9642
      | -12.2748
      | -12.5863
      | -12.8985
      | -13.2113
      | -13.5246
      | -13.8382
      | -14.1519
      | -14.4657
      | -14.7794
      | -15.0928
      | -15.4057
      | -15.7180
      | -16.0296
      | -16.3403
      | -16.6498
      | -16.9582
      | -17.2651
      | -17.5704
      | -17.8739
      | -18.1755
      | -18.4750
      | -18.7722
      | -19.0669
      | -19.3589
      | -19.6481
      | -19.9342
      | -20.2170
      | -20.4964
      | -20.7722
      | -21.0441
      | -21.3119
      | -21.5755
      | -21.8345
      | -22.0889
      | -22.3383
      | -22.5826
      | -22.8216
      | -23.0549
      | -23.2825
      | -23.5040
      | -23.7192
      | -23.9279
      | -24.1298
      | -24.3247
      | -24.5125
      | -24.6927
      | -24.8653
      | -25.0299
      | -25.1863
      | -25.3343
      | -25.4736
      | -25.6040
      | -25.7253
      | -25.8372
      | -25.9395
      | -26.0319
      | -26.1142
      | -26.1863
      | -26.2478
      | -26.2986
      | -26.3385
      | -26.3672
      | -26.3845
      | -26.3903
      | ]
  Steer_angle_right : Lookup_n-D  NumberOfTableDimensions=1  BreakpointsForDimension1=|  Table=|  InternalRulePriority=Speed  RndMeth=Simplest  InputSameDT=on
      BreakpointsForDimension1=|
      | [0
      | 0.014331519
      | 0.057018697
      | 0.127600467
      | 0.225615761
      | 0.350603511
      | 0.50210265
      | 0.679652108
      | 0.882790819
      | 1.111057714
      | 1.363991726
      | 1.64113179
      | 1.942016843
      | 2.266185824
      | 2.613177679
      | 2.982531359
      | 3.373785821
      | 3.786480036
      | 4.220152983
      | 4.674343657
      | 5.148591068
      | 5.642434246
      | 6.155412241
      | 6.687064127
      | 7.236929001
      | 7.804545991
      | 8.389454253
      | 8.991192974
      | 9.609301375
      | 10.24331871
      | 10.89278428
      | 11.55723741
      | 12.23621746
      | 12.92926384
      | 13.63591601
      | 14.35571344
      | 15.08819567
      | 15.83290225
      | 16.58937279
      | 17.35714693
      | 18.13576436
      | 18.92476478
      | 19.72368794
      | 20.53207362
      | 21.34946163
      | 22.17539181
      | 23.00940402
      | 23.85103814
      | 24.69983409
      | 25.55533177
      | 26.41707113
      | 27.28459211
      | 28.15743467
      | 29.03513874
      | 29.91724429
      | 30.80329126
      | 31.69281959
      | 32.5853692
      | 33.48047999
      | 34.37769185
      | 35.27654463
      | 36.17657814
      | 37.07733217
      | 37.97834646
      | 38.87916071
      | 39.77931454
      | 40.67834756
      | 41.57579927
      | 42.47120913
      | 43.36411653
      | 44.25406075
      | 45.14058103
      | 46.0232165
      | 46.90150619
      | 47.77498904
      | 48.6432039
      | 49.5056895
      | 50.36198444
      | 51.21162725
      | 52.05415631
      | 52.88910986
      | 53.71602605
      | 54.53444287
      | 55.3438982
      | 56.14392975
      | 56.93407511
      | 57.71387173
      | 58.48285692
      | 59.24056782
      | 59.98654144
      | 60.72031464
      | 61.44142415
      | 62.14940652
      | 62.84379819
      | 63.52413542
      | 64.18995437
      | 64.84079103
      | 65.47618129
      | 66.09566087
      | 66.6987654
      | 67.28503038
      | 67.85399122
      | 68.4051832
      | 68.93814154
      | 69.45240136
      | 69.94749771
      | 70.4229656
      | 70.87833997
      | 71.31315575
      | 71.72694784
      | 72.11925116
      | 72.48960062
      | 72.83753118
      | 73.16257784
      | 73.46427569
      | 73.74215988
      | 73.9957657
      | 74.22462855
      | 74.42828398
      | 74.60626772
      | 74.75811568
      | 74.883364
      | 74.98154904
      | 75.0522074
      | 75.09487599
      | 75.10909199
      | ]
      Table=|
      | [0.0000
      | -0.0046
      | -0.0183
      | -0.0409
      | -0.0723
      | -0.1124
      | -0.1609
      | -0.2178
      | -0.2828
      | -0.3559
      | -0.4369
      | -0.5255
      | -0.6218
      | -0.7254
      | -0.8364
      | -0.9544
      | -1.0793
      | -1.2110
      | -1.3494
      | -1.4943
      | -1.6454
      | -1.8028
      | -1.9661
      | -2.1353
      | -2.3102
      | -2.4907
      | -2.6765
      | -2.8676
      | -3.0638
      | -3.2649
      | -3.4708
      | -3.6813
      | -3.8963
      | -4.1157
      | -4.3392
      | -4.5668
      | -4.7982
      | -5.0334
      | -5.2721
      | -5.5144
      | -5.7599
      | -6.0085
      | -6.2602
      | -6.5147
      | -6.7720
      | -7.0318
      | -7.2941
      | -7.5586
      | -7.8254
      | -8.0941
      | -8.3647
      | -8.6370
      | -8.9109
      | -9.1862
      | -9.4629
      | -9.7407
      | -10.0196
      | -10.2993
      | -10.5799
      | -10.8610
      | -11.1426
      | -11.4246
      | -11.7067
      | -11.9890
      | -12.2711
      | -12.5531
      | -12.8347
      | -13.1158
      | -13.3963
      | -13.6761
      | -13.9549
      | -14.2327
      | -14.5094
      | -14.7847
      | -15.0586
      | -15.3309
      | -15.6015
      | -15.8701
      | -16.1368
      | -16.4013
      | -16.6636
      | -16.9234
      | -17.1806
      | -17.4350
      | -17.6867
      | -17.9353
      | -18.1807
      | -18.4229
      | -18.6616
      | -18.8967
      | -19.1281
      | -19.3555
      | -19.5790
      | -19.7982
      | -20.0132
      | -20.2236
      | -20.4294
      | -20.6304
      | -20.8265
      | -21.0175
      | -21.2032
      | -21.3836
      | -21.5584
      | -21.7275
      | -21.8908
      | -22.0480
      | -22.1991
      | -22.3438
      | -22.4821
      | -22.6138
      | -22.7386
      | -22.8566
      | -22.9674
      | -23.0710
      | -23.1672
      | -23.2558
      | -23.3367
      | -23.4098
      | -23.4748
      | -23.5317
      | -23.5802
      | -23.6203
      | -23.6517
      | -23.6744
      | -23.6881
      | -23.6928
      | ]
  Subsystem : Subsystem
  Subsystem1 : Subsystem
  Sum : Sum
  Sum1 : Sum
  To Workspace : ToWorkspace  VariableName=Fyf_L  SaveFormat=Timeseries  SampleTime=-1
  To Workspace1 : ToWorkspace  VariableName=Fyr_L  SaveFormat=Timeseries  SampleTime=-1
  To Workspace10 : ToWorkspace  VariableName=alphar_r_L  SaveFormat=Timeseries  SampleTime=-1
  To Workspace13 : ToWorkspace  VariableName=Theta_L  SaveFormat=Timeseries  SampleTime=-1
  To Workspace14 : ToWorkspace  VariableName=Steer_angle_L  SaveFormat=Timeseries  SampleTime=-1
  To Workspace15 : ToWorkspace  VariableName=v_L  SaveFormat=Timeseries  SampleTime=-1
  To Workspace3 : ToWorkspace  VariableName=s_L  SaveFormat=Timeseries  SampleTime=-1
  To Workspace4 : ToWorkspace  VariableName=t_L  SaveFormat=Timeseries  SampleTime=-1
  To Workspace5 : ToWorkspace  VariableName=Steering_rate_L  SaveFormat=Timeseries  SampleTime=-1
  To Workspace7 : ToWorkspace  VariableName=alphaf_l_L  SaveFormat=Timeseries  SampleTime=-1
  To Workspace8 : ToWorkspace  VariableName=alphaf_r_L  SaveFormat=Timeseries  SampleTime=-1
  To Workspace9 : ToWorkspace  VariableName=alphar_l_L  SaveFormat=Timeseries  SampleTime=-1
  Out1 : Outport
  Out2 : Outport  Port=2
  Out3 : Outport  Port=3
  Out4 : Outport  Port=4
  wires:
  Rate Limiter2/1 -> To Workspace9/1, Scope3/1, 2-D Lookup Table1/2
  MATLAB Function1/1(alphaf_l) -> Rate Limiter/1
  MATLAB Function/2(ext) -> Selector5/1, Selector4/1, Selector3/1
  Steer_angle_right/1 -> Gain4/1
  Constant1/1 -> MATLAB Function/4(Fr), MATLAB Function/5(Fl)
  Derivative/1 -> To Workspace5/1
  MATLAB Function1/3(alphar_l) -> Rate Limiter2/1
  Rate Limiter/1 -> To Workspace7/1, Scope1/1, 2-D Lookup Table/2
  Gain1/1 -> Integrator3/1
  Subsystem1/2(normal force on tire rr) -> 2-D Lookup Table3/1
  Selector/1 -> MATLAB Function1/1(Py), Gain/1
  Selector4/1 -> Out2/1
  Sum/1 -> To Workspace/1, MATLAB Function/6(Fyf)
  Steer_angle_left/1 -> Gain3/1
  In2/1 -> Gain5/1
  Subsystem/2(normal force on tire rf) -> 2-D Lookup Table2/1
  2-D Lookup Table/1 -> Sum/1
  2-D Lookup Table2/1 -> Sum/2
  Selector5/1 -> Out3/1
  2-D Lookup Table3/1 -> Sum1/2
  Rate Limiter1/1 -> To Workspace8/1, 2-D Lookup Table2/2, Scope2/1
  Delay/1 -> Selector2/1, Integrator2/1
  Integrator2/1 -> MATLAB Function/1(s), To Workspace3/1, Selector/1, Selector1/1
  Sum1/1 -> To Workspace1/1, MATLAB Function/7(Fyr)
  2-D Lookup Table1/1 -> Sum1/1
  MATLAB Function1/4(alphar_r) -> Rate Limiter3/1
  Selector1/1 -> Gain1/1, MATLAB Function1/2(Pr)
  Subsystem1/1(normal force on tire lr) -> 2-D Lookup Table1/1
  Selector2/1 -> Subsystem1/2(ay), Gain2/1, Subsystem/2(ay)
  Integrator3/1 -> MATLAB Function/2(theta), To Workspace13/1
  Subsystem/1(normal force on tire lf) -> 2-D Lookup Table/1
  Clock/1 -> To Workspace4/1, MATLAB Function/3(t), Subsystem1/1(t), Subsystem/1(t)
  MATLAB Function/1(ds) -> Delay/1
  Gain5/1 -> MATLAB Function/8(u), MATLAB Function1/5(u)
  Selector3/1 -> Out1/1
  MATLAB Function1/5(delta_avg) -> MATLAB Function/9(delta)
  Gain4/1 -> MATLAB Function1/4(delta_r)
  Gain/1 -> To Workspace15/1
  In1/1 -> To Workspace14/1, Derivative/1, Scope/1, Steer_angle_left/1, Steer_angle_right/1
  Gain3/1 -> MATLAB Function1/3(delta_l)
  MATLAB Function1/2(alphaf_r) -> Rate Limiter1/1
  Rate Limiter3/1 -> To Workspace10/1, Scope4/1, 2-D Lookup Table3/2
  Gain2/1 -> Out4/1

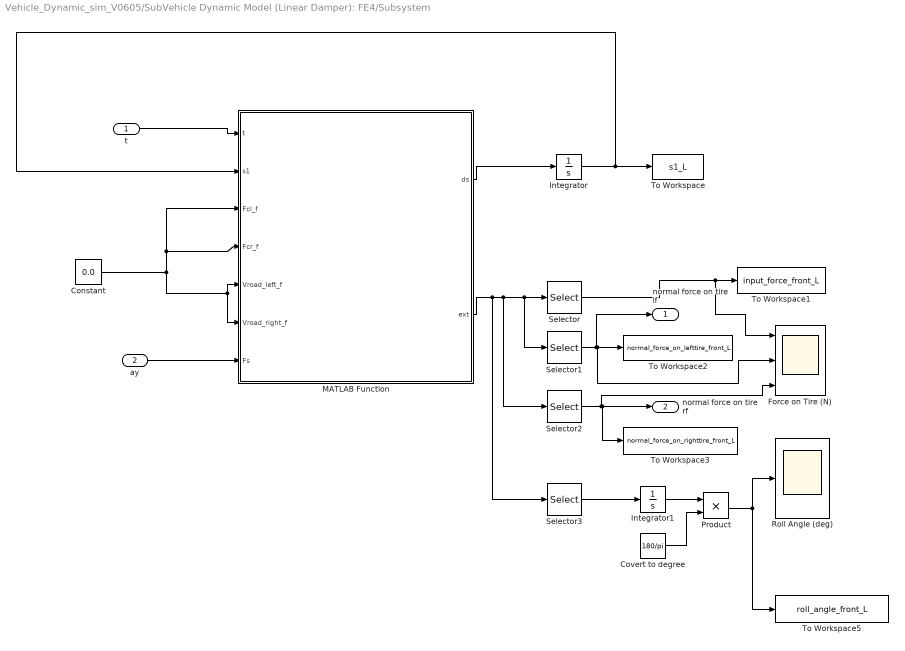
== system Vehicle_Dynamic_sim_V0605/SubVehicle Dynamic Model (Linear Damper): FE4/Subsystem ==
  t : Inport
  ay : Inport  Port=2
  Constant : Constant  Value=0.0
  Covert to degree : Constant  Value=180/pi
  Force on Tire (N) : Scope  NumInputPorts=3
  Integrator : Integrator  InitialCondition=initial_2
  Integrator1 : Integrator
  MATLAB Function : MATLAB Function  TreatAsAtomicUnit=on
  Product : Product
  Roll Angle (deg) : Scope
  Selector : Selector  InputPortWidth=4  IndexOptions=Index vector (dialog)  Indices=[1]  OutputSizes=1
  Selector1 : Selector  InputPortWidth=4  IndexOptions=Index vector (dialog)  Indices=[2]  OutputSizes=1
  Selector2 : Selector  InputPortWidth=4  IndexOptions=Index vector (dialog)  Indices=[3]  OutputSizes=1
  Selector3 : Selector  InputPortWidth=4  IndexOptions=Index vector (dialog)  Indices=[4]  OutputSizes=1
  To Workspace : ToWorkspace  VariableName=s1_L  SaveFormat=Timeseries  SampleTime=-1
  To Workspace1 : ToWorkspace  VariableName=input_force_front_L  SaveFormat=Timeseries  SampleTime=-1
  To Workspace2 : ToWorkspace  VariableName=normal_force_on_lefttire_front_L  SaveFormat=Timeseries  SampleTime=-1
  To Workspace3 : ToWorkspace  VariableName=normal_force_on_righttire_front_L  SaveFormat=Timeseries  SampleTime=-1
  To Workspace5 : ToWorkspace  VariableName=roll_angle_front_L  SaveFormat=Timeseries  SampleTime=-1
  normal force on tire lf : Outport
  normal force on tire rf : Outport  Port=2
  wires:
  t/1 -> MATLAB Function/1(t)
  MATLAB Function/1(ds) -> Integrator/1
  Integrator/1 -> MATLAB Function/2(s1), To Workspace/1
  MATLAB Function/2(ext) -> Selector3/1, Selector2/1, Selector1/1, Selector/1
  Selector1/1 -> normal force on tire lf/1, Force on Tire (N)/2, To Workspace2/1
  Selector2/1 -> normal force on tire rf/1, To Workspace3/1, Force on Tire (N)/3
  Constant/1 -> MATLAB Function/4(Fcr_f), MATLAB Function/3(Fcl_f), MATLAB Function/6(Vroad_right_f), MATLAB Function/5(Vroad_left_f)
  Selector3/1 -> Integrator1/1
  Covert to degree/1 -> Product/2
  Integrator1/1 -> Product/1
  Product/1 -> To Workspace5/1, Roll Angle (deg)/1
  ay/1 -> MATLAB Function/7(Fs)
  Selector/1 -> Force on Tire (N)/1, To Workspace1/1
